simulink model "DAC"  (R2023b)
settings: Solver=VariableStepAuto  StartTime=0.0  StopTime=10.0  RelTol=1e-3
settings Model: Creator=ycheb  LastModifiedBy=ycheb

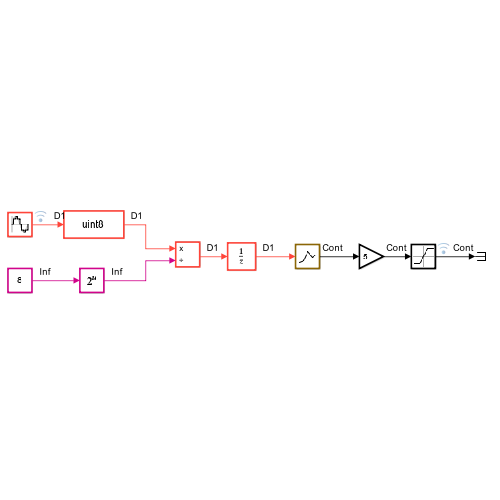
[thumbnail: Simulink's stored preview of the top-level diagram]
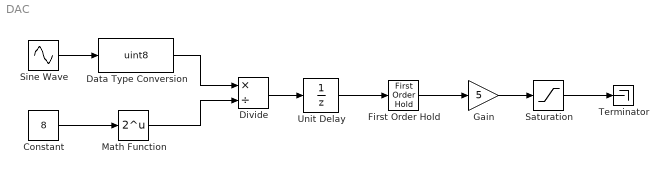
== system DAC ==
  Constant : Constant  Value=8
  Data Type Conversion : DataTypeConversion  OutDataTypeStr=uint8  SaturateOnIntegerOverflow=off  RndMeth=Floor
  Divide : Product  Inputs=*/
  First Order Hold : FirstOrderHold  ErrorTolerance=inf
  Gain : Gain  Gain=5
  Math Function : Math  Operator=2^u
  Saturation : Saturate  UpperLimit=5  LowerLimit=0
  Sine Wave : Sin  Amplitude=2^8/2  Bias=2^8/2  Frequency=10  Phase=-pi /2  SampleTime=1e-4
  Terminator : Terminator
  Unit Delay : UnitDelay  SampleTime=-1  HasFrameUpgradeWarning=on
  wires:
  Sine Wave/1 -> Data Type Conversion/1
  Data Type Conversion/1 -> Divide/1
  Constant/1 -> Math Function/1
  Math Function/1 -> Divide/2
  Gain/1 -> Saturation/1
  Divide/1 -> Unit Delay/1
  Unit Delay/1 -> First Order Hold/1
  First Order Hold/1 -> Gain/1
  Saturation/1 -> Terminator/1
